simulink model "Mooventure2016_Rev5"  (Simulink 7.7)
settings: Solver=FixedStepDiscrete  StartTime=0.0  StopTime=10  RelTol=1e-3
PreLoadFcn:
  | try, eval([bdroot '_setup']); catch, eval('model_setup', ''); end
InitFcn:
  | try, eval([bdroot '_setup']); catch, eval('model_setup', ''); end
undefined symbols (not defined in the file): ECM, H1, motohawk_build_version, motohawk_trunc_name, motohawk_vardec_config_group, motohawk_vardec_path, xD
libraries: MotoHawk_lib x976, motohawk_control_primitives_lib x41, simulink x27, motohawk_annotations_lib x3
(part 10 of 16)

== system Mooventure2016_Rev5/Foreground/Inputs/Battery_Inputs/SOC Filter ==
  In1 : Inport
  First Order Low Pass (Tunable) : Subsystem  mask(First-Order Low-Pass Filter (Tunable)){nam='SOCFilt', samp_time=10, group=motohawk_vardec_path(gcb)}
      mask prompts: nam "Name"; samp_time "Sample Time"; group "MotoTune Group String"
      mask help:
      | Discrete first-order low-pass filter, with calibratable time-constant.
      |
      | If 'Sample Time' is -1, then extra code and RAM will be generated to dynamically calculate dt.
      mask Display:
      | patch([0 0 1 1], [0 0.075 0.075 0], [230/255 0/255 0/255])
      | patch([0 0 1 1], [0.025 0.05 0.05 0.025], [150/255 0/255 0/255])
      | patch([0 0 1 1], [0 0.025 0.025 0], [0/255 0/255 0/255])
      | 
      | disp('1st-Order\nLow Pass');
  Out1 : Outport
  wires:
  In1/1 -> First Order Low Pass (Tunable)/1(in)
  First Order Low Pass (Tunable)/1(out) -> Out1/1

== system Mooventure2016_Rev5/Foreground/Inputs/Battery_Inputs/Voltage Filter ==
  In1 : Inport
  First Order Low Pass (Tunable) : Subsystem  mask(First-Order Low-Pass Filter (Tunable)){nam='VFilt', samp_time=10, group=motohawk_vardec_path(gcb)}
      mask prompts: nam "Name"; samp_time "Sample Time"; group "MotoTune Group String"
      mask help:
      | Discrete first-order low-pass filter, with calibratable time-constant.
      |
      | If 'Sample Time' is -1, then extra code and RAM will be generated to dynamically calculate dt.
      mask Display:
      | patch([0 0 1 1], [0 0.075 0.075 0], [230/255 0/255 0/255])
      | patch([0 0 1 1], [0.025 0.05 0.05 0.025], [150/255 0/255 0/255])
      | patch([0 0 1 1], [0 0.025 0.025 0], [0/255 0/255 0/255])
      | 
      | disp('1st-Order\nLow Pass');
  Out1 : Outport
  wires:
  In1/1 -> First Order Low Pass (Tunable)/1(in)
  First Order Low Pass (Tunable)/1(out) -> Out1/1

== system Mooventure2016_Rev5/Foreground/Inputs/Cruise Control/Button Delay 1 ==
  In1 : Inport
  Time : Inport  Port=2
  Logical Operator : Logic  AllPortsSameDT=off  OutDataTypeStr=boolean
  Relational Operator : RelationalOperator  OutDataTypeStr=boolean
  Time Since Enabled (With Input)4 : motohawk_control_primitives_lib/Time Since Enabled (With Input)1  SystemSampleTime=-1  nam='ButtonDelay1'  samp_time=-1  init=0  upperlim=3600*24
  Out1 : Outport
  wires:
  In1/1 -> Time Since Enabled (With Input)4/1, Logical Operator/1
  Time Since Enabled (With Input)4/1 -> Relational Operator/1
  Time/1 -> Relational Operator/2
  Relational Operator/1 -> Logical Operator/2
  Logical Operator/1 -> Out1/1

== system Mooventure2016_Rev5/Foreground/Inputs/Cruise Control/Button Delay 2 ==
  In1 : Inport
  Time : Inport  Port=2
  Logical Operator : Logic  AllPortsSameDT=off  OutDataTypeStr=boolean
  Relational Operator : RelationalOperator  OutDataTypeStr=boolean
  Time Since Enabled (With Input)4 : motohawk_control_primitives_lib/Time Since Enabled (With Input)1  SystemSampleTime=-1  nam='ButtonDelay2'  samp_time=-1  init=0  upperlim=3600*24
  Out1 : Outport
  wires:
  In1/1 -> Time Since Enabled (With Input)4/1, Logical Operator/1
  Time Since Enabled (With Input)4/1 -> Relational Operator/1
  Time/1 -> Relational Operator/2
  Relational Operator/1 -> Logical Operator/2
  Logical Operator/1 -> Out1/1

== system Mooventure2016_Rev5/Foreground/Inputs/Cruise Control/Button Delay 3 ==
  In1 : Inport
  Time : Inport  Port=2
  Logical Operator : Logic  AllPortsSameDT=off  OutDataTypeStr=boolean
  Relational Operator : RelationalOperator  OutDataTypeStr=boolean
  Time Since Enabled (With Input)4 : motohawk_control_primitives_lib/Time Since Enabled (With Input)1  SystemSampleTime=-1  nam='ButtonDelay3'  samp_time=-1  init=0  upperlim=3600*24
  Out1 : Outport
  wires:
  In1/1 -> Time Since Enabled (With Input)4/1, Logical Operator/1
  Time Since Enabled (With Input)4/1 -> Relational Operator/1
  Time/1 -> Relational Operator/2
  Relational Operator/1 -> Logical Operator/2
  Logical Operator/1 -> Out1/1

== system Mooventure2016_Rev5/Foreground/Inputs/Cruise Control/Button Delay 4 ==
  In1 : Inport
  Time : Inport  Port=2
  Logical Operator : Logic  AllPortsSameDT=off  OutDataTypeStr=boolean
  Relational Operator : RelationalOperator  OutDataTypeStr=boolean
  Time Since Enabled (With Input)4 : motohawk_control_primitives_lib/Time Since Enabled (With Input)1  SystemSampleTime=-1  nam='ButtonDelay4'  samp_time=-1  init=0  upperlim=3600*24
  Out1 : Outport
  wires:
  In1/1 -> Time Since Enabled (With Input)4/1, Logical Operator/1
  Time Since Enabled (With Input)4/1 -> Relational Operator/1
  Time/1 -> Relational Operator/2
  Relational Operator/1 -> Logical Operator/2
  Logical Operator/1 -> Out1/1

== system Mooventure2016_Rev5/Foreground/Inputs/Cruise Control/Button Delay 5 ==
  In1 : Inport
  Time : Inport  Port=2
  Logical Operator : Logic  AllPortsSameDT=off  OutDataTypeStr=boolean
  Relational Operator : RelationalOperator  OutDataTypeStr=boolean
  Time Since Enabled (With Input)4 : motohawk_control_primitives_lib/Time Since Enabled (With Input)1  SystemSampleTime=-1  nam='ButtonDelay5'  samp_time=-1  init=0  upperlim=3600*24
  Out1 : Outport
  wires:
  In1/1 -> Time Since Enabled (With Input)4/1, Logical Operator/1
  Time Since Enabled (With Input)4/1 -> Relational Operator/1
  Time/1 -> Relational Operator/2
  Relational Operator/1 -> Logical Operator/2
  Logical Operator/1 -> Out1/1

== system Mooventure2016_Rev5/Foreground/Inputs/IPT CAN Inputs/Subsystem ==
  In1 : Inport
  In2 : Inport  Port=2
  In3 : Inport  Port=3
  In4 : Inport  Port=4
  In5 : Inport  Port=5
  In6 : Inport  Port=6
  In7 : Inport  Port=7
  Bus Creator : BusCreator  Inputs=7
  Out1 : Outport
  wires:
  In1/1 -> Bus Creator/1
  In2/1 -> Bus Creator/2
  In3/1 -> Bus Creator/3
  In4/1 -> Bus Creator/4
  In5/1 -> Bus Creator/5
  In6/1 -> Bus Creator/6
  In7/1 -> Bus Creator/7
  Bus Creator/1 -> Out1/1  "ID 260 IPT Status 2"

== system Mooventure2016_Rev5/Foreground/Outputs/Coolant Outputs/Delay 1 ==
  Signal : Inport
  Threshold : Inport  Port=2
  Logical Operator : Logic  AllPortsSameDT=off  OutDataTypeStr=boolean
  Relational Operator3 : RelationalOperator  OutDataTypeStr=boolean
  Time Since Enabled (With Input)4 : motohawk_control_primitives_lib/Time Since Enabled (With Input)1  SystemSampleTime=-1  nam='Heat1Timer'  samp_time=-1  init=0  upperlim=3600*24
  Signal Out : Outport
  wires:
  Signal/1 -> Time Since Enabled (With Input)4/1, Logical Operator/2
  Time Since Enabled (With Input)4/1 -> Relational Operator3/1
  Threshold/1 -> Relational Operator3/2
  Relational Operator3/1 -> Logical Operator/1
  Logical Operator/1 -> Signal Out/1

== system Mooventure2016_Rev5/Foreground/Outputs/Coolant Outputs/Delay 2 ==
  Signal : Inport
  Threshold : Inport  Port=2
  Logical Operator : Logic  AllPortsSameDT=off  OutDataTypeStr=boolean
  Relational Operator3 : RelationalOperator  OutDataTypeStr=boolean
  Time Since Enabled (With Input)4 : motohawk_control_primitives_lib/Time Since Enabled (With Input)1  SystemSampleTime=-1  nam='Heat2Timer'  samp_time=-1  init=0  upperlim=3600*24
  Signal Out : Outport
  wires:
  Signal/1 -> Time Since Enabled (With Input)4/1, Logical Operator/2
  Time Since Enabled (With Input)4/1 -> Relational Operator3/1
  Threshold/1 -> Relational Operator3/2
  Relational Operator3/1 -> Logical Operator/1
  Logical Operator/1 -> Signal Out/1

== system Mooventure2016_Rev5/Foreground/Outputs/Coolant Outputs/Delay 3 ==
  Signal : Inport
  Threshold : Inport  Port=2
  Logical Operator : Logic  AllPortsSameDT=off  OutDataTypeStr=boolean
  Relational Operator3 : RelationalOperator  OutDataTypeStr=boolean
  Time Since Enabled (With Input)4 : motohawk_control_primitives_lib/Time Since Enabled (With Input)1  SystemSampleTime=-1  nam='Heat3Timer'  samp_time=-1  init=0  upperlim=3600*24
  Signal Out : Outport
  wires:
  Signal/1 -> Time Since Enabled (With Input)4/1, Logical Operator/2
  Time Since Enabled (With Input)4/1 -> Relational Operator3/1
  Threshold/1 -> Relational Operator3/2
  Relational Operator3/1 -> Logical Operator/1
  Logical Operator/1 -> Signal Out/1

== system Mooventure2016_Rev5/Foreground/Outputs/Coolant Outputs/Delay 4 ==
  Signal : Inport
  Threshold : Inport  Port=2
  Logical Operator : Logic  AllPortsSameDT=off  OutDataTypeStr=boolean
  Relational Operator3 : RelationalOperator  OutDataTypeStr=boolean
  Time Since Enabled (With Input)4 : motohawk_control_primitives_lib/Time Since Enabled (With Input)1  SystemSampleTime=-1  nam='Heat4Timer'  samp_time=-1  init=0  upperlim=3600*24
  Signal Out : Outport
  wires:
  Signal/1 -> Time Since Enabled (With Input)4/1, Logical Operator/2
  Time Since Enabled (With Input)4/1 -> Relational Operator3/1
  Threshold/1 -> Relational Operator3/2
  Relational Operator3/1 -> Logical Operator/1
  Logical Operator/1 -> Signal Out/1

== system Mooventure2016_Rev5/Foreground/Outputs/DistributionBox/Heat Check ==
  Logical Operator : Logic  Operator=OR  Inputs=4  AllPortsSameDT=off  OutDataTypeStr=boolean
  Out1 : Outport
  wires:
  [Heat1] -> Logical Operator/1
  [Heat2] -> Logical Operator/2
  [Heat3] -> Logical Operator/3
  [Heat4] -> Logical Operator/4
  Logical Operator/1 -> Out1/1

== system Mooventure2016_Rev5/Foreground/Outputs/Driver Ouputs/Enabled Subsystem ==
  Enable : EnablePort
  Bar Chart Reset : Stateflow chart  TreatAsAtomicUnit=on
  motohawk_calibration2 : MotoHawk_lib/Calibration & Probing Blocks/motohawk_calibration  nam='Temp_Flash'  val=1200  storage=Calibration  show_more=on  name_source=Use Parameter  data_type=double  read_level=1  write_level=1  ovr_cals=on  view_as=Number  enum_struct={'Disabled', 'Enabled'}  vector_style=Wide Row  use_help_units=off  help=''  units=''  use_header_enum=off  row_header_enum={}  col_header_enum={}  use_min_max=off  min_val=-inf  max_val=inf  use_precision=on  precision=''  gain=0.05  offset=0  exp=1  use_mototune_group=off  mototune_group=motohawk_vardec_path(gcb)
  Out1 : Outport
  wires:
  motohawk_calibration2/1 -> Bar Chart Reset/1(delay)
  Bar Chart Reset/1(write) -> Out1/1

== system Mooventure2016_Rev5/Foreground/Outputs/Driver Ouputs/Integrator ==
  note: Discrete Integrator,
      | with output and state saturation.
  In : Inport
  Rst : Inport  Port=2
  IC : Inport  Port=3
  Min : Inport  Port=4
  Max : Inport  Port=5
  Data Type Conversion : DataTypeConversion  OutDataTypeStr=boolean  RndMeth=Zero
  Product : Product  SaturateOnIntegerOverflow=on  InputSameDT=on  OutDataTypeStr=Inherit: Same as first input
  Saturation : motohawk_control_primitives_lib/Saturation  SystemSampleTime=-1
  Switch1 : Switch  Threshold=1  ZeroCross=off  SaturateOnIntegerOverflow=on  InputSameDT=on
  motohawk_delta_time : MotoHawk_lib/Extra Development Blocks/motohawk_delta_time  samp_time=-1  init_val=0  mode=Seconds (double)
  Out : Outport
  wires:
  IC/1 -> Switch1/1
  Max/1 -> Saturation/3
  Min/1 -> Saturation/2
  Data Type Conversion/1 -> Switch1/2
  Rst/1 -> Data Type Conversion/1
  Product/1 -> Saturation/1
  In/1 -> Product/1
  motohawk_delta_time/1 -> Product/2
  Switch1/1 -> Out/1
  Saturation/1 -> Switch1/3
